simulink subsystem "clipping_Dmin"  (R2024a)
settings: Solver=VariableStepAuto  StartTime=0.0  StopTime=10.0  RelTol=1e-3
undefined symbols (not defined in the file or in its folder): D_min
settings Model: Creator=Peter  LastModifiedBy=Peter

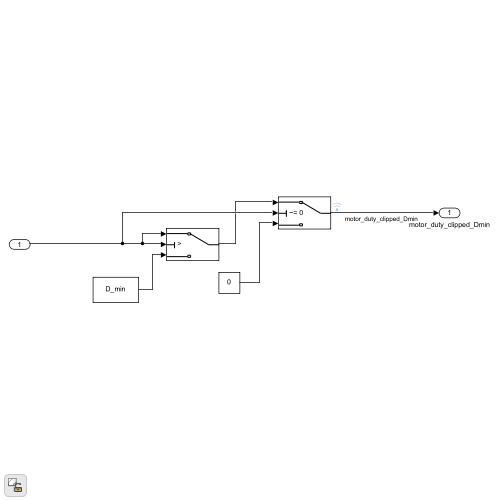
[thumbnail: Simulink's stored preview of the top-level diagram]
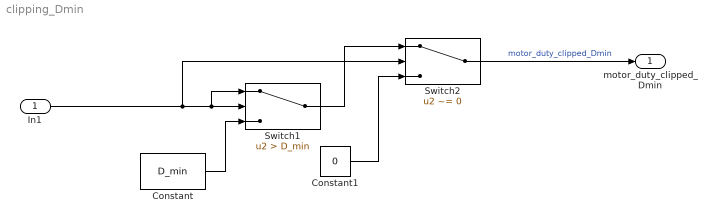
== system clipping_Dmin ==
  In1 : Inport
  Constant : Constant  Value=D_min  OutDataTypeStr=single
  Constant1 : Constant  Value=0  OutDataTypeStr=single
  Switch1 : Switch  Criteria=u2 > Threshold  Threshold=D_min  OutDataTypeStr=single  SaturateOnIntegerOverflow=off  InputSameDT=off
  Switch2 : Switch  Criteria=u2 ~= 0  OutDataTypeStr=single  SaturateOnIntegerOverflow=off  InputSameDT=off
  motor_duty_clipped_Dmin : Outport
  wires:
  In1/1 -> Switch1/1, Switch1/2, Switch2/2
  Switch1/1 -> Switch2/1
  Constant1/1 -> Switch2/3
  Switch2/1 -> motor_duty_clipped_Dmin/1  "motor_duty_clipped_Dmin"
  Constant/1 -> Switch1/3
